simulink model "doublMassControl"  (R2016b)
settings: Solver=VariableStepAuto  StartTime=0.0  StopTime=0.4  FixedStep=2e-4  RelTol=1e-3
values from neighbouring files (symbols this model uses):
  denGp = [m1*m2 0 (m1+m2)*k 0 0]    [doubleMassInit.m]
  denominator = denominator{1}    [doubleMassInit.m]    (also in mainFeedbackTuning.m)
  numerator = numerator{1}    [doubleMassInit.m]    (also in mainFeedbackTuning.m)
  numGp = k    (= 64481415.4205)    [doubleMassInit.m]
  snapCoef = mean(tempErr)*dcgain(sysc)/mean(tempSnap)    [calCoef.m]    (also in doubleMassInit.m = 6.62981724598e-07)
  Ts = 1/fs    (= 0.0001)    [doubleMassInit.m]    (also in mainFeedbackTuning.m)
libraries: model_controller x3, simulink x1
settings Model: Creator=Dai Luyao  LastModifiedBy=Dai Luyao

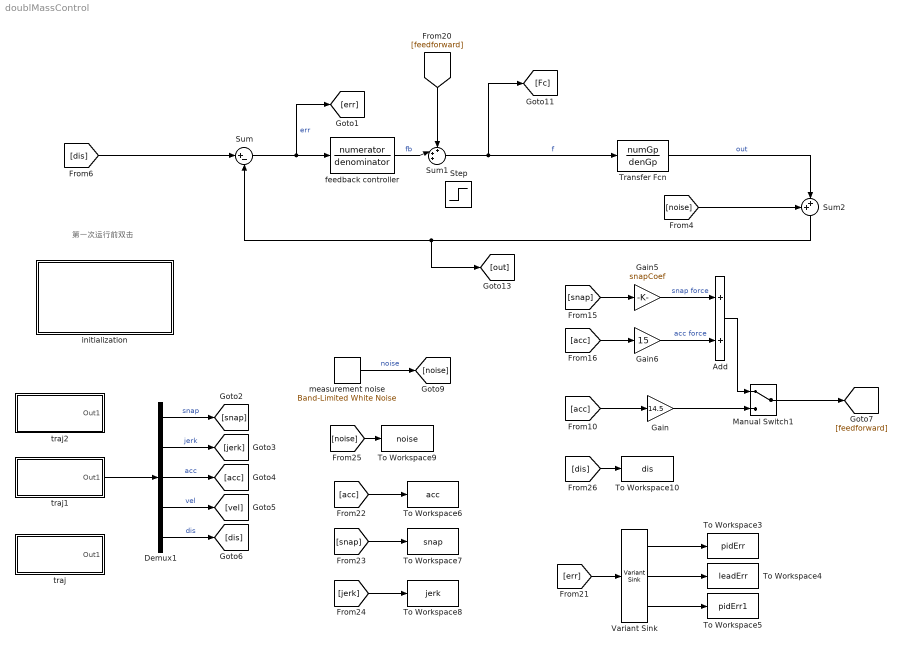
== system doublMassControl ==
  note: 第一次运行前双击
  Add : Sum
  Demux1 : Demux  Outputs=5
  Gain : Gain  Gain=14.5
  Gain5 : Gain  Gain=snapCoef
  Gain6 : Gain  Gain=15
  Manual Switch1 : ManualSwitch
  Step : Step  Time=0  After=0.2  SampleTime=0
  Sum : Sum  Inputs=|+-
  Sum1 : Sum  Inputs=+++|
  Sum2 : Sum  Inputs=++|
  To Workspace10 : ToWorkspace  VariableName=dis  SaveFormat=Structure With Time  SampleTime=-1
  To Workspace3 : ToWorkspace  VariableName=pidErr  SaveFormat=Structure With Time  SampleTime=-1
  To Workspace4 : ToWorkspace  VariableName=leadErr  SaveFormat=Structure With Time  SampleTime=-1
  To Workspace5 : ToWorkspace  VariableName=pidErr1  SaveFormat=Structure With Time  SampleTime=-1
  To Workspace6 : ToWorkspace  VariableName=acc  SaveFormat=Structure With Time  SampleTime=-1
  To Workspace7 : ToWorkspace  VariableName=snap  SaveFormat=Structure With Time  SampleTime=-1
  To Workspace8 : ToWorkspace  VariableName=jerk  SaveFormat=Structure With Time  SampleTime=-1
  To Workspace9 : ToWorkspace  VariableName=noise  SaveFormat=Structure With Time  SampleTime=-1
  Transfer Fcn : TransferFcn  Numerator=numGp  Denominator=denGp
  Variant Sink : VariantSink
  feedback controller : TransferFcn  Numerator=numerator  Denominator=denominator
  initialization : Subsystem
      settings: OpenFcn=doubleMassInit;  MoveFcn=edit doubleMassInit;
  measurement noise : simulink/Sources/Band-Limited White Noise  Cov=noisePower  Ts=Ts  seed=[23000]
  traj : Subsystem  BlockChoice=4th order traj
      link override 4th order traj: v=0.5  x=0.1  j=500
      settings: AttributesFormatString=%<BlockChoice>  TemplateBlock=model_controller/Profile Generators/traj  MemberBlocks=2th order traj,3rd order traj,4th order traj,step
  traj1 : Subsystem  BlockChoice=4th order traj
      link override 4th order traj: v=0.5  x=0.1  j=500
      settings: AttributesFormatString=%<BlockChoice>  TemplateBlock=model_controller/Profile Generators/traj  MemberBlocks=2th order traj,3rd order traj,4th order traj,step
  traj2 : Subsystem  BlockChoice=4th order traj
      link override 4th order traj: v=0.6  x=0.1  j=700  d=20000
      settings: AttributesFormatString=%<BlockChoice>  TemplateBlock=model_controller/Profile Generators/traj  MemberBlocks=2th order traj,3rd order traj,4th order traj,step
  wires:
  Sum/1 -> feedback controller/1, [err]  "err"
  feedback controller/1 -> Sum1/2  "fb"
  Sum1/1 -> Transfer Fcn/1, [Fc]  "f"
  measurement noise/1 -> [noise]  "noise"
  Transfer Fcn/1 -> Sum2/2  "out"
  [noise] -> Sum2/1
  Sum2/1 -> [out], Sum/2
  Demux1/1 -> [snap]  "snap"
  Demux1/2 -> [jerk]  "jerk"
  Demux1/3 -> [acc]  "acc"
  Demux1/4 -> [vel]  "vel"
  Demux1/5 -> [dis]  "dis"
  [acc] -> Gain/1
  [snap] -> Gain5/1
  [acc] -> Gain6/1
  Gain5/1 -> Add/1  "snap force"
  Gain6/1 -> Add/2  "acc force"
  Add/1 -> Manual Switch1/1
  Gain/1 -> Manual Switch1/2
  Manual Switch1/1 -> [feedforward]
  [err] -> Variant Sink/1
  Variant Sink/1 -> To Workspace3/1
  Variant Sink/2 -> To Workspace4/1
  Variant Sink/3 -> To Workspace5/1
  [acc] -> To Workspace6/1
  [snap] -> To Workspace7/1
  [jerk] -> To Workspace8/1
  traj1/1(Out1) -> Demux1/1
  [noise] -> To Workspace9/1
  [dis] -> To Workspace10/1
  [dis] -> Sum/1
  [feedforward] -> Sum1/1

== system doublMassControl/initialization ==

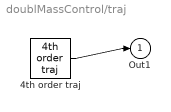
== system doublMassControl/traj ==
  4th order traj : model_controller/Profile Generators/4th order traj  t0=0  x=0.1  v=0.5  a=10  j=500  d=64000  Ts=0
  Out1 : Outport
  wires:
  4th order traj/1 -> Out1/1

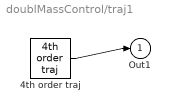
== system doublMassControl/traj1 ==
  4th order traj : model_controller/Profile Generators/4th order traj  t0=0  x=0.1  v=0.5  a=10  j=500  d=64000  Ts=0
  Out1 : Outport
  wires:
  4th order traj/1 -> Out1/1

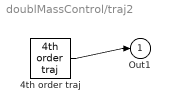
== system doublMassControl/traj2 ==
  4th order traj : model_controller/Profile Generators/4th order traj  t0=0  x=0.1  v=0.6  a=10  j=700  d=20000  Ts=0
  Out1 : Outport
  wires:
  4th order traj/1 -> Out1/1
